simulink model "checkNegativeModel"  (R2018a)
settings: Solver=VariableStepAuto  StartTime=startTimesmlk  StopTime=0.045  RelTol=1e-3
values from neighbouring files (symbols this model uses):
  N_neg = rscale(ss_neg.A,ss_neg.B,ss_neg.C,ss_neg.D,K_neg)    [check_NegativeModelGAM.m]
  startTime = time(1)    [check_NegativeModelGAM.m]
  sys_negKAL = ss(kest_neg.A,kest_neg.B,kest_neg.C,kest_neg.D,Ts)    [check_NegativeModelGAM.m]
undefined symbols (not defined in the file or in its folder): K_neg, ss_neg, x0_neg
settings Model: Creator=dori  LastModifiedBy=dori

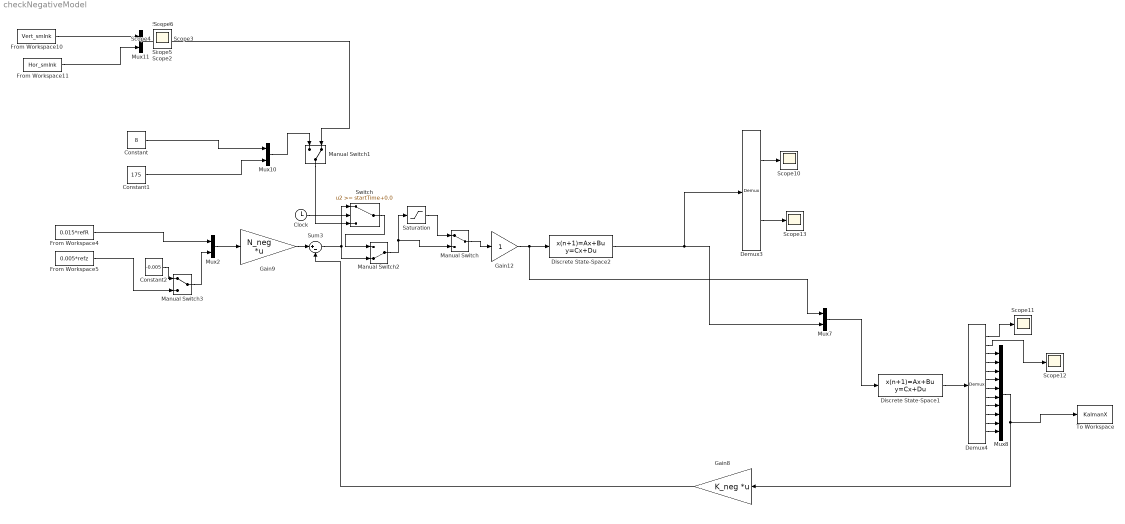
== system checkNegativeModel ==
  Clock : Clock
  Constant : Constant  Value=8
  Constant1 : Constant  Value=175
  Constant2 : Constant  Value=-0.005
  Demux3 : Demux  Outputs=2
  Demux4 : Demux  Outputs=12
  Discrete State-Space1 : DiscreteStateSpace  A=sys_negKAL.A  B=sys_negKAL.B  C=sys_negKAL.C  D=sys_negKAL.D  InitialCondition=x0_neg  SampleTime=100e-6
  Discrete State-Space2 : DiscreteStateSpace  A=ss_neg.A  B=ss_neg.B  C=ss_neg.C  D=ss_neg.D  InitialCondition=x0_neg  SampleTime=100e-6
  From Workspace10 : FromWorkspace  VariableName=Vert_smlnk
  From Workspace11 : FromWorkspace  VariableName=Hor_smlnk
  From Workspace4 : FromWorkspace  VariableName=0.015*refR  SampleTime=0
  From Workspace5 : FromWorkspace  VariableName=0.005*refz  SampleTime=0
  Gain12 : Gain
  Gain8 : Gain  Gain=K_neg  Multiplication=Matrix(K*u)
  Gain9 : Gain  Gain=N_neg  Multiplication=Matrix(K*u)
  Manual Switch : ManualSwitch
  Manual Switch1 : ManualSwitch  CurrentSetting=0
  Manual Switch2 : ManualSwitch  CurrentSetting=0
  Manual Switch3 : ManualSwitch
  Mux{2,7,10..11} (4 alike) : Mux  Inputs=2
  Mux8 : Mux  Inputs=10
  Saturation : Saturate  UpperLimit=[300,175]  LowerLimit=[-300,-175]
  Scope{,1..6,10..13} (11 alike) : Scope
  Sum3 : Sum  Inputs=|+-
  Switch : Switch  Threshold=startTime+0.0
  To Workspace : ToWorkspace  VariableName=KalmanX  SaveFormat=Structure With Time  SampleTime=-1
  wires:
  Mux11/1 -> Manual Switch1/2
  Saturation/1 -> Manual Switch/1
  Discrete State-Space1/1 -> Demux4/1
  Demux3/1 -> Scope10/1
  Demux4/10 -> Mux8/8
  Demux3/2 -> Scope13/1
  From Workspace4/1 -> Mux2/1
  Mux7/1 -> Discrete State-Space1/1
  Demux4/2 -> Scope12/1
  Mux10/1 -> Manual Switch1/1
  Demux4/7 -> Mux8/5
  Demux4/1 -> Scope11/1
  Sum3/1 -> Manual Switch2/2, Switch/1
  Gain12/1 -> Mux7/1, Discrete State-Space2/1
  Mux8/1 -> To Workspace/1, Gain8/1
  Gain9/1 -> Sum3/1
  Demux4/12 -> Mux8/10
  Gain8/1 -> Sum3/2
  Demux4/5 -> Mux8/3
  Demux4/11 -> Mux8/9
  Manual Switch/1 -> Gain12/1
  Demux4/3 -> Mux8/1
  Discrete State-Space2/1 -> Demux3/1, Mux7/2
  Constant1/1 -> Mux10/2
  Manual Switch1/1 -> Switch/3
  From Workspace11/1 -> Mux11/2
  Clock/1 -> Switch/2
  Mux2/1 -> Gain9/1
  Demux4/9 -> Mux8/7
  Demux4/4 -> Mux8/2
  Constant/1 -> Mux10/1
  Switch/1 -> Manual Switch2/1
  Demux4/8 -> Mux8/6
  Demux4/6 -> Mux8/4
  From Workspace10/1 -> Mux11/1
  Manual Switch2/1 -> Manual Switch/2, Saturation/1
  From Workspace5/1 -> Manual Switch3/2
  Manual Switch3/1 -> Mux2/2
  Constant2/1 -> Manual Switch3/1
